simulink model "FunnelController"  (R2024b)
settings: Solver=FixedStepAuto  StartTime=0.0  StopTime=inf  RelTol=1e-3  EnableMultiTasking=on
undefined symbols (not defined in the file or in its folder): Ts
libraries: arduinomotorcarrierlib x4, simulink x1, eeGeneralControl x1, dspstat3 x1, arduinosensorlib x1
settings Model: SimulationMode=external  ExtModeTrigDuration=2  Creator=ammar  LastModifiedBy=niek-
settings SolverCC: AutoInsertRateTranBlk=on
settings OptimizationCC: EnhancedBackFolding=on  PassReuseOutputArgsAs=Individual arguments  ZeroExternalMemoryAtStartup=off  ZeroInternalMemoryAtStartup=off  MaxStackSize=64  OptimizeBlockOrder=speed  DifferentSizesBufferReuse=on  EfficientTunableParamExpr=on
settings DebuggingCC: ParameterTunabilityLossMsg=error  UnderSpecifiedDimensionMsg=warning
settings HardwareCC: ProdBitPerPointer=32  ProdBitPerSizeT=32  ProdBitPerPtrDiffT=32  ProdLargestAtomicInteger=Long  ProdLargestAtomicFloat=Double  ProdWordSize=32  ProdHWDeviceType=ARM Compatible->ARM Cortex  UseEmbeddedCoderFeatures=off  UseSimulinkCoderFeatures=off
settings SFSimCC: MATLABDynamicMemAlloc=off
settings RTWCC: Description=Embedded Coder  SystemTargetFile=ert.tlc  HardwareBoard=Arduino Nano 33 IoT  TemplateMakefile=ert_default_tmf  Toolchain=Arduino ARM  BuildConfiguration=Faster Runs
settings CodeAppCC: ForceParamTrailComments=on  IgnoreCustomStorageClasses=off  OperatorAnnotations=on  SimulinkDataObjDesc=on  SFDataObjDesc=on  InsertBlockDesc=on
settings ERTTargetCC: SupportContinuousTime=on  SupportNonInlinedSFcns=on  SupportVariableSizeSignals=on  ExtModeTransport=2  ExtModeStaticAlloc=on  ExtModeAutomaticAllocSize=off  ExtModeStaticAllocSize=8192  ExtModeMexFile=ext_xcp  ExtModeIntrfLevel=Level2 - Open  InlinedParameterPlacement=Hierarchical

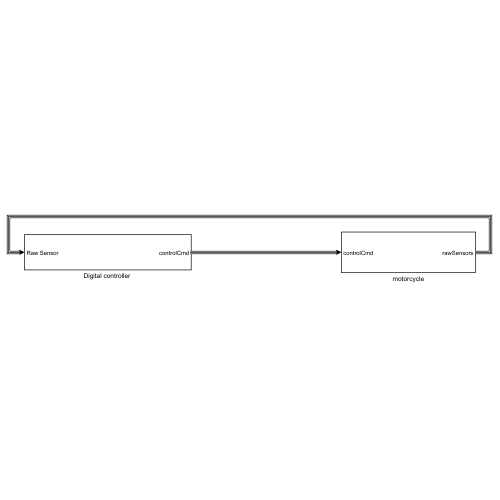
[thumbnail: Simulink's stored preview of the top-level diagram]
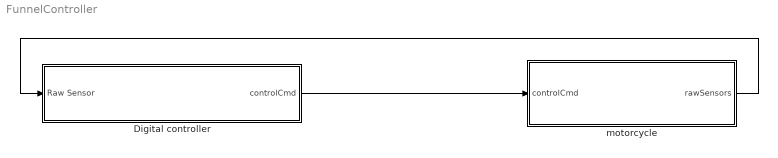
== system FunnelController ==
  "Digital controller " : Subsystem
  motorcycle : Subsystem
  wires:
  "Digital controller "/1(controlCmd) -> motorcycle/1(controlCmd)
  motorcycle/1(rawSensors) -> "Digital controller "/1(Raw Sensor)

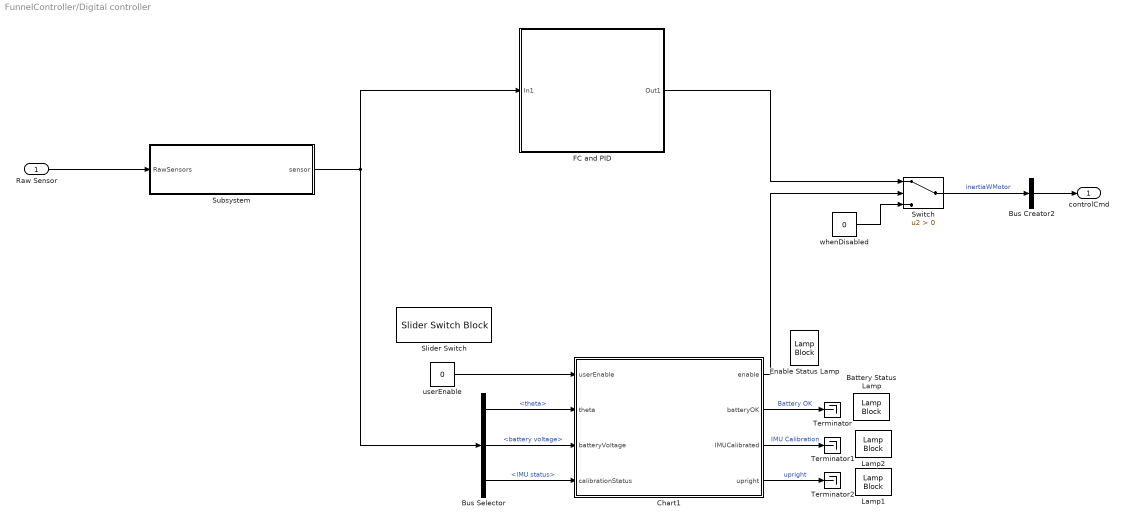
== system FunnelController/Digital controller  ==
  Raw Sensor : Inport
  Battery Status Lamp : LampBlock  LabelPosition=Hide
  Bus Creator2 : BusCreator  Inputs=1
  Bus Selector : BusSelector  OutputSignals=theta,battery voltage,IMU status
  Chart1 : Stateflow chart  TreatAsAtomicUnit=on
  Enable Status Lamp : LampBlock  LabelPosition=Hide
  FC and PID : Subsystem
  Lamp1 : LampBlock  LabelPosition=Hide
  Lamp2 : LampBlock  LabelPosition=Hide
  Slider Switch : SliderSwitchBlock
      settings: Values={{'Off', 'On'}, [0 1]}
  Subsystem : Subsystem
  Switch : Switch  Criteria=u2 > Threshold  SaturateOnIntegerOverflow=off  InputSameDT=off
  Terminator : Terminator
  Terminator1 : Terminator
  Terminator2 : Terminator
  userEnable : Constant  Value=0  SampleTime=0.01
  whenDisabled : Constant  Value=0  SampleTime=Ts
  controlCmd : Outport
  wires:
  Raw Sensor/1 -> Subsystem/1(RawSensors)
  Bus Selector/3 -> Chart1/4(calibrationStatus)  "<IMU status>"
  Bus Selector/2 -> Chart1/3(batteryVoltage)  "<battery voltage>"
  userEnable/1 -> Chart1/1(userEnable)
  Bus Selector/1 -> Chart1/2(theta)  "<theta>"
  Chart1/3(IMUCalibrated) -> Terminator1/1  "IMU Calibration"
  Chart1/2(batteryOK) -> Terminator/1  "Battery OK"
  Chart1/4(upright) -> Terminator2/1  "upright"
  Subsystem/1(sensor) -> Bus Selector/1, FC and PID/1(In1)
  whenDisabled/1 -> Switch/3
  FC and PID/1(Out1) -> Switch/1
  Chart1/1(enable) -> Switch/2
  Bus Creator2/1 -> controlCmd/1
  Switch/1 -> Bus Creator2/1  "inertiaWMotor"

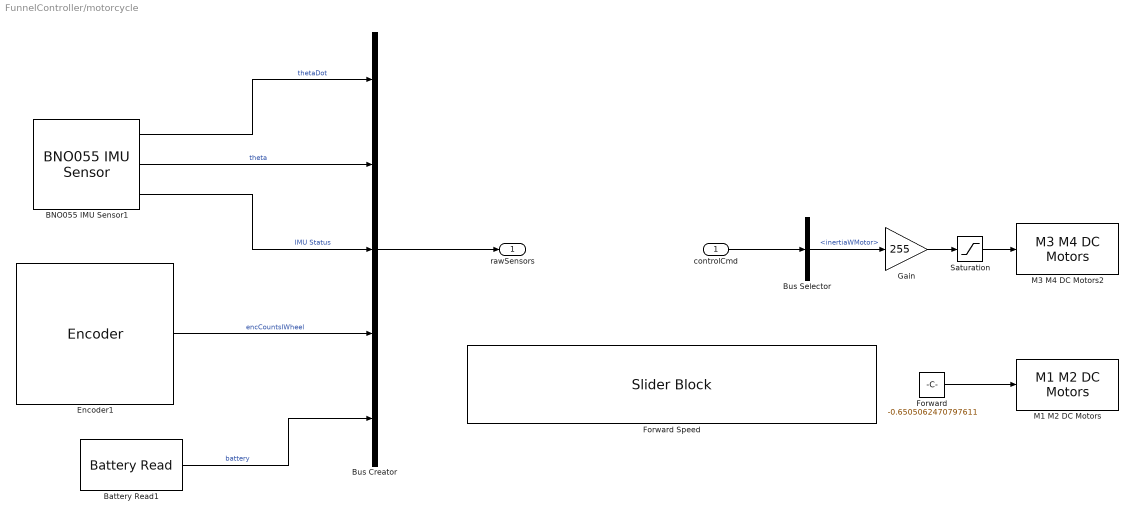
== system FunnelController/motorcycle ==
  controlCmd : Inport
  BNO055 IMU Sensor1 : arduinosensorlib/BNO055 IMU Sensor  I2CModule=0  SlaveAddress=0x28  OperationMode=Fusion  Accel=off  AngularRate=on  MagField=off  EulerAngles=on  Quat=off  LinearAccel=off  GravityVector=off  Status=on  Timestamp=off  AccelRange=4G  AccelBW=62.5 Hz  GyroRange=2000 dps  GyroBW=32 Hz  MagODR=10 Hz  spf=1  SampleTime=Ts  blockPlatform=ARDUINO  QueueSizeFactor=1
      settings: SourceProductName=Sensors
  Battery Read1 : arduinomotorcarrierlib/Battery Read  SlaveAddress=uint8( hex2dec( '66' ) )  blockPlatform=ARDUINO  SampleTime=Ts
      settings: SourceProductName=Arduino Motor Carrier
  Bus Creator : BusCreator  Inputs=5
  Bus Selector : BusSelector  OutputSignals=inertiaWMotor
  Encoder1 : arduinomotorcarrierlib/Encoder  SlaveAddress=uint8( hex2dec( '66' ) )  blockPlatform=ARDUINO  Encoder=1  ShowSpeed=off  ResetOption=on  SampleTime=Ts
      settings: SourceProductName=Arduino Motor Carrier
  Forward : Constant  Value=-0.6505062470797611
  Forward Speed : SliderBlock  ScaleMin=-100
  Gain : Gain  Gain=255
  M1 M2 DC Motors : arduinomotorcarrierlib/M1 M2 DC Motors  SlaveAddress=uint8( hex2dec( '66' ) )  blockPlatform=ARDUINO  MotorNumber=M2  MotorCarrierPWMFreq=100
      settings: SourceProductName=Arduino Motor Carrier
  M3 M4 DC Motors2 : arduinomotorcarrierlib/M3 M4 DC Motors  MotorNumber=M3  forwardPinNumber=3  reversePinNumber=2
      settings: SourceProductName=Arduino Motor Carrier
  Saturation : Saturate  UpperLimit=200  LowerLimit=-200
  rawSensors : Outport
  wires:
  controlCmd/1 -> Bus Selector/1
  BNO055 IMU Sensor1/1 -> Bus Creator/1  "thetaDot"
  BNO055 IMU Sensor1/2 -> Bus Creator/2  "theta"
  BNO055 IMU Sensor1/3 -> Bus Creator/3  "IMU Status"
  Battery Read1/1 -> Bus Creator/5  "battery"
  Encoder1/1 -> Bus Creator/4  "encCountsIWheel"
  Bus Creator/1 -> rawSensors/1
  Bus Selector/1 -> Gain/1  "<inertiaWMotor>"
  Gain/1 -> Saturation/1
  Saturation/1 -> M3 M4 DC Motors2/1
  Forward/1 -> M1 M2 DC Motors/1

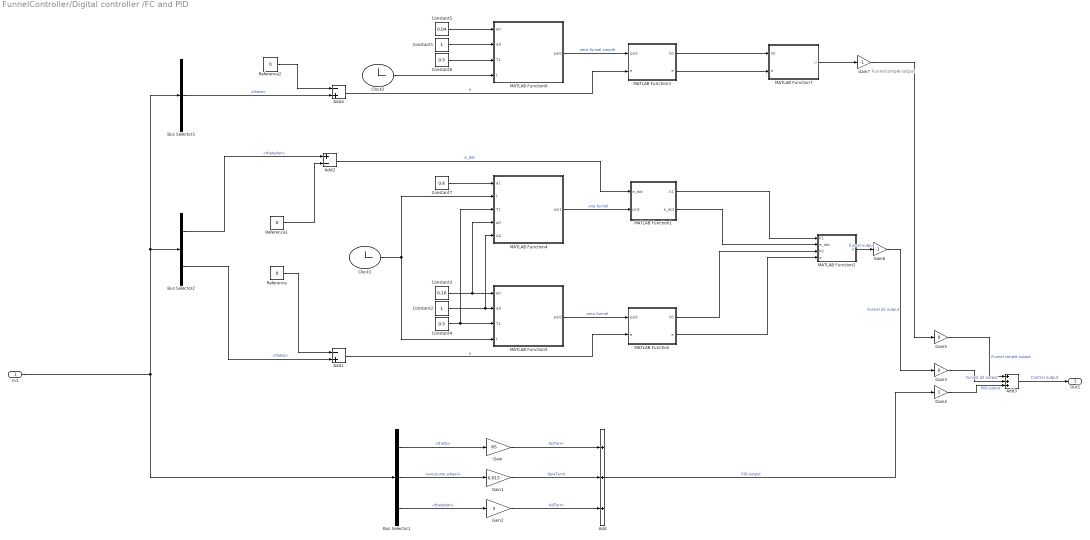
== system FunnelController/Digital controller /FC and PID ==
  note: Funnel simple output
  In1 : Inport
  Add : Sum  Inputs=+++
  Add1 : Sum  Inputs=-+
  Add2 : Sum  Inputs=+-
  Add3 : Sum  Inputs=+++
  Add4 : Sum  Inputs=-+
  Bus Selector1 : BusSelector  OutputSignals=theta,encounts wheel,thetadot
  Bus Selector2 : BusSelector  OutputSignals=thetadot,theta
  Bus Selector3 : BusSelector  OutputSignals=theta
  Clock1 : Clock
  Clock2 : Clock
  Constant1 : Constant
  Constant2 : Constant
  Constant3 : Constant  Value=0.16
  Constant4 : Constant  Value=0.5
  Constant5 : Constant  Value=0.04
  Constant6 : Constant  Value=0.5
  Constant7 : Constant  Value=0.6
  Gain : Gain  Gain=65
  Gain1 : Gain  Gain=0.015
  Gain2 : Gain  Gain=5
  Gain3 : Gain  Gain=0
  Gain4 : Gain
  Gain5 : Gain  Gain=0
  Gain6 : Gain  Gain=-1
  Gain7 : Gain  Gain=-1
  MATLAB Function : MATLAB Function  TreatAsAtomicUnit=on
  MATLAB Function1 : MATLAB Function  TreatAsAtomicUnit=on
  MATLAB Function2 : MATLAB Function  TreatAsAtomicUnit=on
  MATLAB Function3 : MATLAB Function  TreatAsAtomicUnit=on
  MATLAB Function4 : MATLAB Function  TreatAsAtomicUnit=on
  MATLAB Function5 : MATLAB Function  TreatAsAtomicUnit=on
  MATLAB Function6 : MATLAB Function  TreatAsAtomicUnit=on
  MATLAB Function7 : MATLAB Function  TreatAsAtomicUnit=on
  Reference : Constant  Value=0
  Reference1 : Constant  Value=0
  Reference2 : Constant  Value=0
  Out1 : Outport
  wires:
  Add3/1 -> Out1/1  "Control output"
  Gain3/1 -> Add3/2  "Funnel d2 output"
  Gain/1 -> Add/1  "KpTerm"
  Bus Selector1/1 -> Gain/1  "<theta>"
  Add/1 -> Gain4/1  "PID output"
  Gain1/1 -> Add/2  "KpwTerm"
  Gain2/1 -> Add/3  "KdTerm"
  Bus Selector1/3 -> Gain2/1  "<thetadot>"
  Constant7/1 -> MATLAB Function4/1(a1)
  Clock1/1 -> MATLAB Function5/4(t), MATLAB Function4/2(t)
  Constant2/1 -> MATLAB Function4/5(A0), MATLAB Function5/2(A0)
  MATLAB Function5/1(psi0) -> MATLAB Function/1(psi0)  "zero funnel"
  Bus Selector2/1 -> Add2/1  "<thetadot>"
  MATLAB Function1/1(k1) -> MATLAB Function2/1(k1)
  Reference1/1 -> Add2/2
  Constant4/1 -> MATLAB Function4/3(T1), MATLAB Function5/3(T1)
  MATLAB Function/1(k0) -> MATLAB Function2/3(k0)
  Add2/1 -> MATLAB Function1/1("e_dot ")  "e_dot"
  Constant3/1 -> MATLAB Function4/4(a0), MATLAB Function5/1(a0)
  MATLAB Function/2(e) -> MATLAB Function2/4(e)
  MATLAB Function2/1(u) -> Gain6/1  "funnel output"
  Bus Selector2/2 -> Add1/2  "<theta>"
  Add1/1 -> MATLAB Function/2("e ")  "e"
  MATLAB Function4/1(psi1) -> MATLAB Function1/2(psi1)  "one funnel"
  MATLAB Function1/2(e_dot) -> MATLAB Function2/2(e_dot)
  Gain4/1 -> Add3/3  "PID output"
  Reference/1 -> Add1/1
  Reference2/1 -> Add4/1
  Add4/1 -> MATLAB Function3/2("e ")  "e"
  Bus Selector3/1 -> Add4/2  "<theta>"
  MATLAB Function3/2(e) -> MATLAB Function7/2(e)
  Constant5/1 -> MATLAB Function6/1(a0)
  MATLAB Function3/1(k0) -> MATLAB Function7/1(k0)
  Constant6/1 -> MATLAB Function6/3(T1)
  MATLAB Function6/1(psi0) -> MATLAB Function3/1(psi0)  "zero funnel simple"
  Constant1/1 -> MATLAB Function6/2(A0)
  Clock2/1 -> MATLAB Function6/4(t)
  In1/1 -> Bus Selector3/1, Bus Selector2/1, Bus Selector1/1
  MATLAB Function7/1(u) -> Gain7/1
  Gain5/1 -> Add3/1  "Funnel simple output"
  Bus Selector1/2 -> Gain1/1  "<encounts wheel>"
  Gain6/1 -> Gain3/1  "Funnel d2 output"
  Gain7/1 -> Gain5/1

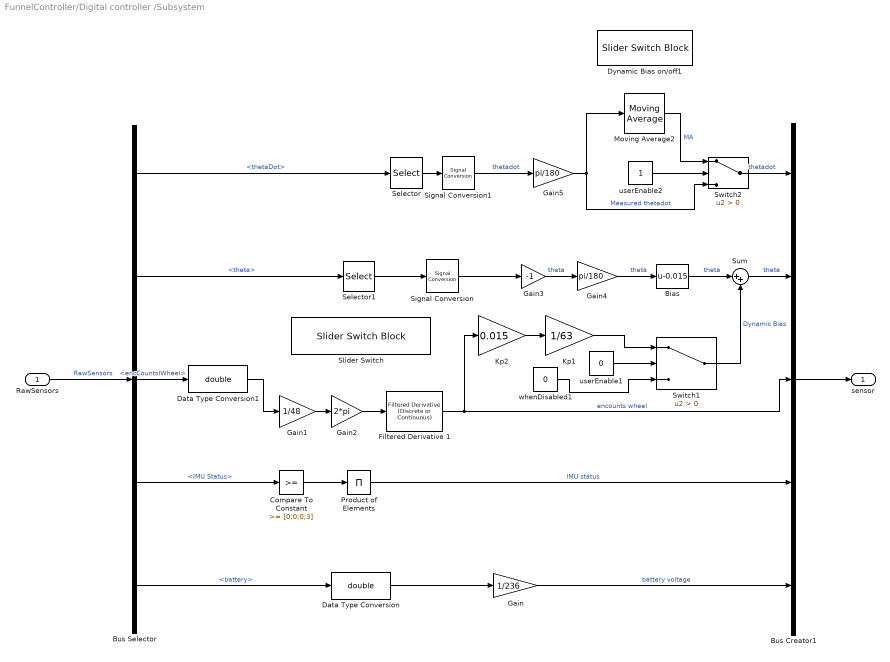
== system FunnelController/Digital controller /Subsystem ==
  RawSensors : Inport  SampleTime=0.01
  Bias : Bias  Bias=-0.015  SaturateOnIntegerOverflow=off
  Bus Creator1 : BusCreator  Inputs=5
  Bus Selector : BusSelector  OutputSignals=thetaDot,theta,encCountsIWheel,IMU Status,battery
  Compare To Constant : simulink/Logic and Bit Operations/Compare To Constant  relop=>=  const=[0;0;0;3]  OutDataTypeStr=boolean
  Data Type Conversion : DataTypeConversion  OutDataTypeStr=double  SaturateOnIntegerOverflow=off  RndMeth=Floor
  Data Type Conversion1 : DataTypeConversion  OutDataTypeStr=double  SaturateOnIntegerOverflow=off  RndMeth=Floor
  Dynamic Bias on/off1 : SliderSwitchBlock
      settings: Values={{'Off', 'On'}, [0 1]}
  Filtered Derivative 1 : eeGeneralControl/Filtered Derivative (Discrete or Continuous)  K=1  T=0.1  B=inf  A=-inf  minRatio=10  init_option=Inherited from block input  x0=0  Ts=0.01
      settings: LibrarySourceBlock=|
      | ee_sl_lib/General Control/Filtered Derivative
      | (Discrete or Continuous)
  Gain : Gain  Gain=1/236
  Gain1 : Gain  Gain=1/48
  Gain2 : Gain  Gain=2*pi
  Gain3 : Gain  Gain=-1
  Gain4 : Gain  Gain=pi/180
  Gain5 : Gain  Gain=pi/180
  Kp1 : Gain  Gain=1/63
  Kp2 : Gain  Gain=0.015
  Moving Average2 : dspstat3/Moving Average  Method=Sliding window  ForgettingFactorPort=off  SpecifyWindowLength=on  WindowLength=3  OverlapLength=2  AllowArbitraryInputLength=off  ForgettingFactor=0.9  SimulateUsing=Interpreted execution
  Product of Elements : Product  Inputs=*
  Selector : Selector  InputPortWidth=3  IndexOptions=Index vector (dialog)  Indices=[2]  OutputSizes=1
  Selector1 : Selector  InputPortWidth=3  IndexOptions=Index vector (dialog)  Indices=[2]  OutputSizes=1
  Signal Conversion : SignalConversion  OverrideOpt=off
  Signal Conversion1 : SignalConversion  OverrideOpt=off
  Slider Switch : SliderSwitchBlock
      settings: Values={{'Off', 'On'}, [0 1]}
  Sum : Sum  Inputs=|++
  Switch1 : Switch  Criteria=u2 > Threshold  SaturateOnIntegerOverflow=off  InputSameDT=off
  Switch2 : Switch  Criteria=u2 > Threshold  SaturateOnIntegerOverflow=off  InputSameDT=off
  userEnable1 : Constant  Value=0  SampleTime=Ts
  userEnable2 : Constant  SampleTime=Ts
  whenDisabled1 : Constant  Value=0  SampleTime=Ts
  sensor : Outport  SampleTime=0.01
  wires:
  Gain1/1 -> Gain2/1
  Filtered Derivative 1/1 -> Bus Creator1/3, Kp2/1  "encounts wheel"
  Gain2/1 -> Filtered Derivative 1/1
  Bus Selector/5 -> Data Type Conversion/1  "<battery>"
  Signal Conversion1/1 -> Gain5/1  "thetadot"
  Product of Elements/1 -> Bus Creator1/4  "IMU status"
  Bus Selector/3 -> Data Type Conversion1/1  "<encCountsIWheel>"
  Data Type Conversion1/1 -> Gain1/1
  Data Type Conversion/1 -> Gain/1
  Bus Selector/2 -> Selector1/1  "<theta>"
  Bus Creator1/1 -> sensor/1
  Gain3/1 -> Gain4/1  "theta"
  Gain/1 -> Bus Creator1/5  "battery voltage"
  RawSensors/1 -> Bus Selector/1  "RawSensors"
  Bus Selector/4 -> Compare To Constant/1  "<IMU Status>"
  Bus Selector/1 -> Selector/1  "<thetaDot>"
  Selector/1 -> Signal Conversion1/1
  Compare To Constant/1 -> Product of Elements/1
  Signal Conversion/1 -> Gain3/1
  Selector1/1 -> Signal Conversion/1
  Switch2/1 -> Bus Creator1/1  "thetadot"
  Gain4/1 -> Bias/1  "theta"
  Bias/1 -> Sum/1  "theta"
  Sum/1 -> Bus Creator1/2  "theta"
  Gain5/1 -> Moving Average2/1, Switch2/3  "Measured thetadot"
  Moving Average2/1 -> Switch2/1  "MA"
  userEnable2/1 -> Switch2/2
  userEnable1/1 -> Switch1/2
  whenDisabled1/1 -> Switch1/3
  Switch1/1 -> Sum/2  "Dynamic Bias"
  Kp1/1 -> Switch1/1
  Kp2/1 -> Kp1/1

== matlab function FunnelController/Digital controller /FC and PID/MATLAB Function ==
  data: k0 output; e output; psi0 input; e input
function [k0,e]=   K_value(psi0, e)

k0 = 1 / (psi0 - abs(e)) ;

end

== matlab function FunnelController/Digital controller /FC and PID/MATLAB Function1 ==
  data: k1 output; e_dot input; psi1 input; e_dot output
function [k1,e_dot] =   K_value(e_dot,psi1)

k1 = 1 / (psi1 - abs(e_dot)) ;

end

== matlab function FunnelController/Digital controller /FC and PID/MATLAB Function2 ==
  data: u output; k1 input; e_dot input; k0 input; e input
function u = u_value(k1,e_dot, k0,e)

u = (-k0^2) * e - k1 * e_dot;

end

== matlab function FunnelController/Digital controller /FC and PID/MATLAB Function3 ==
  data: k0 output; e output; psi0 input; e input
function [k0,e]=   K_value(psi0, e)

k0 = 1 / (psi0 - abs(e)) ;

end

== matlab function FunnelController/Digital controller /FC and PID/MATLAB Function4 ==
  data: a1 input; t input; T1 input; a0 input; A0 input; psi1 output
function psi1 = k_value(a1, t, T1, a0, A0)

psi1 = (A0 - a0) / T1 * exp(-t / T1) + a1;

end

== matlab function FunnelController/Digital controller /FC and PID/MATLAB Function5 ==
  data: a0 input; A0 input; T1 input; t input; psi0 output
function psi0  = k_value(a0, A0, T1, t)

psi0 = (A0 - a0) * exp(-t / T1) + a0;

end

== matlab function FunnelController/Digital controller /FC and PID/MATLAB Function6 ==
  data: a0 input; A0 input; T1 input; t input; psi0 output
function psi0  = k_value(a0, A0, T1, t)

psi0 = (A0 - a0) * exp(-t / T1) + a0;

end

== matlab function FunnelController/Digital controller /FC and PID/MATLAB Function7 ==
  data: u output; k0 input; e input
function u = u_simple(k0,e)

u = -k0 * e;

end

== stateflow chart FunnelController/Digital controller /Chart1 ==
  state checkFallen [parallel]
    settings: executionOrder=1
    state fallen
      entry: upright = false
    state standing
      entry: upright = true
    (default) -> fallen
    fallen -> standing : [abs(theta) <pi*13.4/180]
    standing -> fallen : [abs(theta) > pi*13.4/180]
  state checkIMUCalib [parallel]
    settings: executionOrder=2
    state imuNotCalibrated
      entry:
      IMUCalibrated = false;
    state imuCalibrated
      entry:
      IMUCalibrated = true;
    (default) -> imuNotCalibrated
    imuNotCalibrated -> imuCalibrated : [calibrationStatus == true]
  state checkBattery [parallel]
    settings: executionOrder=3
    state batteryNotCharged
      entry:
      batteryOK = false;
    state batteryCharged
      entry:
      batteryOK = true;
    (default) -> batteryNotCharged
    batteryCharged -> batteryNotCharged : [batteryVoltage < 3.0]
    batteryNotCharged -> batteryCharged : [batteryVoltage >= 3.0]
  state calculateEnable [parallel]
    settings: executionOrder=4
    state disableControl
      entry: enable = false
    state enableControl
      entry: enable = true
    (default) -> disableControl
    disableControl -> enableControl : [userEnable&& batteryOK && IMUCalibrated && upright]
    enableControl -> disableControl : [not(userEnable) || not(batteryOK) || not(IMUCalibrated) || not(upright)]
  data: userEnable input; theta input; enable output; batteryVoltage input; calibrationStatus input; batteryOK output; IMUCalibrated output; upright output
